simulink model "sim_PID"  (R2019b)
settings: Solver=VariableStepAuto  StartTime=0.0  StopTime=30  RelTol=1e-3
values from neighbouring files (symbols this model uses):
  F = 3    [values.m]
  LA = (uN*alfa_5*T_prima-rho*Cd*vN*A)/m    (= -0.00793822342637)    [values.m]
  LB = alfa_5*Tm*(1-beta*(alfa_5*vN/wm -1)^2)/m    (= 1.26917363265)    [values.m]
  t_c = -g*cos(theta_N)/(LB) *(slope_grades*pi/180)    [values.m]
  Ts = 0.2    [Transformacion_bilineal.m]    (also in values.m)
  uN = (m*g*Cr+rho*Cd*A*(vN^2)/2)/(alfa_5*T_alpha_n_v)    (= 0.145774916245)    [values.m]
  vN = 16.7    [values.m]
undefined symbols (not defined in the file or in its folder): k_CC, k_CD, k_GD, p_CC, p_CD, p_GD, z_CC, z_CD, z_GD
settings Model: Creator=Esteban  LastModifiedBy=Esteban

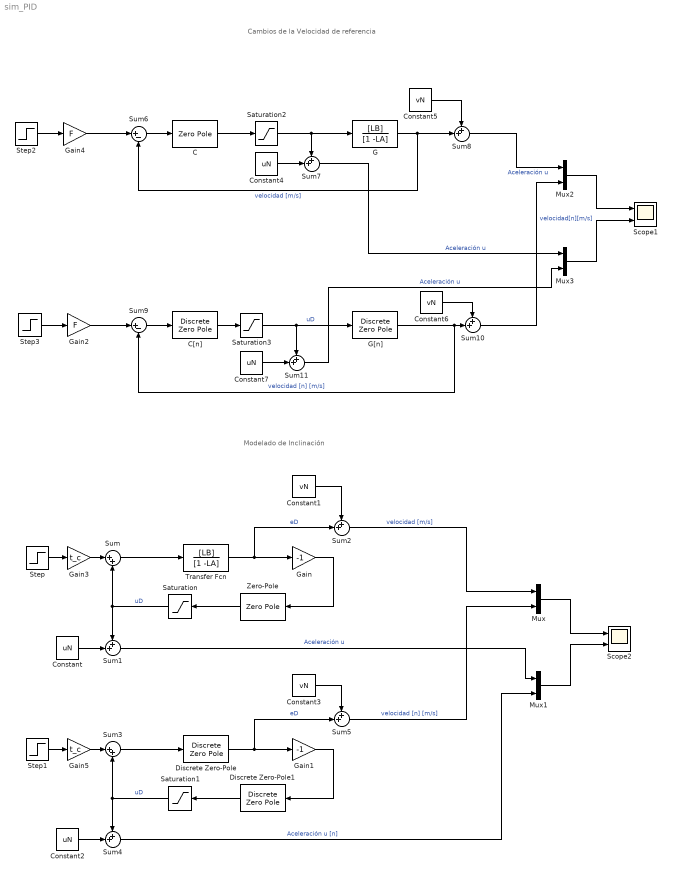
== system sim_PID ==
  note: Cambios de la Velocidad de referencia
  note: Modelado de Inclinación
  C : ZeroPole  Zeros=[z_CC{:,1}]  Poles=[p_CC{:,1}]  Gain=[k_CC]
  C[n] : DiscreteZeroPole  Zeros=[z_CD{:,1}]  Poles=[p_CD{:,1}]  Gain=k_CD  SampleTime=Ts
  Constant{,2,4,7} (4 alike) : Constant  Value=uN
  Constant{1,3,5..6} (4 alike) : Constant  Value=vN
  Discrete Zero-Pole : DiscreteZeroPole  Zeros=[z_GD{:,1}]  Poles=[p_GD{:,1}]  Gain=k_GD  SampleTime=Ts
  Discrete Zero-Pole1 : DiscreteZeroPole  Zeros=[z_CD{:,1}]  Poles=[p_CD{:,1}]  Gain=k_CD  SampleTime=Ts
  G : TransferFcn  Numerator=[LB]  Denominator=[1 -LA]
  G[n] : DiscreteZeroPole  Zeros=[z_GD{:,1}]  Poles=[p_GD{:,1}]  Gain=k_GD  SampleTime=Ts
  Gain : Gain  Gain=-1
  Gain1 : Gain  Gain=-1
  Gain2 : Gain  Gain=F
  Gain3 : Gain  Gain=t_c
  Gain4 : Gain  Gain=F
  Gain5 : Gain  Gain=t_c
  Mux{,1..3} (4 alike) : Mux  Inputs=2
  Saturation{,1..3} (4 alike) : Saturate  UpperLimit=1-uN  LowerLimit=-uN
  Scope1 : Scope  NumInputPorts=2
  Scope2 : Scope  NumInputPorts=2
  Step : Step  SampleTime=0
  Step1 : Step  SampleTime=Ts
  Step2 : Step  SampleTime=0
  Step3 : Step  SampleTime=Ts
  Sum : Sum  Inputs=|++
  Sum{1..2,4..5,7..8,10..11} (8 alike) : Sum  Inputs=++|
  Sum3 : Sum  Inputs=|++
  Sum6 : Sum  Inputs=|+-
  Sum9 : Sum  Inputs=|+-
  Transfer Fcn : TransferFcn  Numerator=[LB]  Denominator=[1 -LA]
  Zero-Pole : ZeroPole  Zeros=[z_CC{:,1}]  Poles=[p_CC{:,1}]  Gain=[k_CC]
  wires:
  Sum/1 -> Transfer Fcn/1
  Transfer Fcn/1 -> Sum2/2, Gain/1  "eD"
  Zero-Pole/1 -> Saturation/1
  Step/1 -> Gain3/1
  Gain/1 -> Zero-Pole/1
  Constant/1 -> Sum1/2
  Sum1/1 -> Mux1/1  "Aceleración u"
  Constant1/1 -> Sum2/1
  Sum2/1 -> Mux/1  "velocidad [m/s]"
  Saturation/1 -> Sum1/1, Sum/2  "uD"
  Constant3/1 -> Sum5/1
  Sum4/1 -> Mux1/2  "Aceleración u [n]"
  Gain1/1 -> Discrete Zero-Pole1/1
  Constant2/1 -> Sum4/2
  Sum5/1 -> Mux/2  "velocidad [n] [m/s]"
  Sum3/1 -> Discrete Zero-Pole/1
  Step1/1 -> Gain5/1
  Discrete Zero-Pole/1 -> Sum5/2, Gain1/1  "eD"
  Saturation1/1 -> Sum4/1, Sum3/2  "uD"
  Discrete Zero-Pole1/1 -> Saturation1/1
  Mux/1 -> Scope2/1
  Mux1/1 -> Scope2/2
  Mux2/1 -> Scope1/1
  Mux3/1 -> Scope1/2
  Sum9/1 -> C[n]/1
  Step3/1 -> Gain2/1
  G[n]/1 -> Sum10/2, Sum9/2  "velocidad [n] [m/s]"
  G/1 -> Sum8/2, Sum6/2  "velocidad [m/s]"
  Sum6/1 -> C/1
  Constant4/1 -> Sum7/2
  C/1 -> Saturation2/1
  C[n]/1 -> Saturation3/1
  Gain3/1 -> Sum/1
  Gain5/1 -> Sum3/1
  Step2/1 -> Gain4/1
  Saturation2/1 -> Sum7/1, G/1
  Saturation3/1 -> Sum11/1, G[n]/1  "uD"
  Gain4/1 -> Sum6/1
  Sum7/1 -> Mux3/1  "Aceleración u"
  Sum8/1 -> Mux2/1  "Aceleración u"
  Constant5/1 -> Sum8/1
  Gain2/1 -> Sum9/1
  Constant7/1 -> Sum11/2
  Sum11/1 -> Mux3/2  "Aceleración u"
  Constant6/1 -> Sum10/1
  Sum10/1 -> Mux2/2  "velocidad[n][m/s]"
